simulink model "dof"  (R2024b)
settings: Solver=VariableStepAuto  StartTime=0.0  StopTime=200  RelTol=1e-3
libraries: aerolibanim x1, shared6dof x1, aerolibatmos2 x1, aerolibasang x1
settings Model: Creator=isaac  LastModifiedBy=Isaac

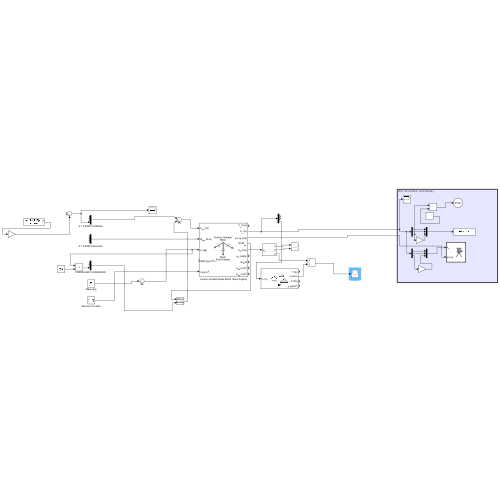
[thumbnail: Simulink's stored preview of the top-level diagram]
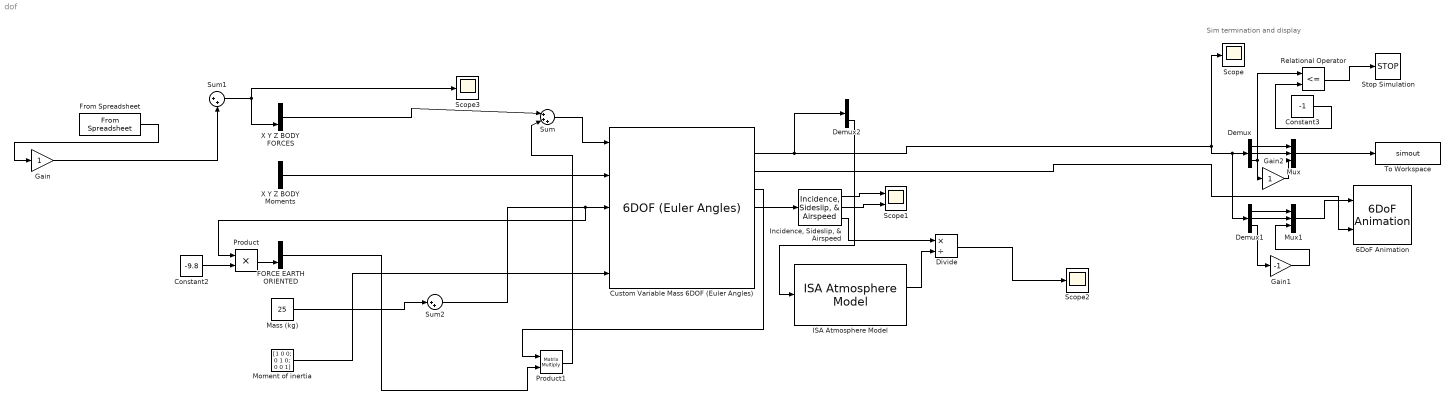
== system dof ==
  note: Sim termination and display
  6DoF Animation : aerolibanim/6DoF Animation  u1=[-5000 5000 -5000 5000 -15000 0]  u2=0.1  u3=50  u4=[4000 0 -5000]  u5=Fly alongside  u6=[20000 5000 -30000]  u7=10  u8=on
  Constant2 : Constant  Value=-9.8
  Constant3 : Constant  Value=-1
  Custom Variable Mass 6DOF (Euler Angles) : shared6dof/6DOF (Euler Angles)  units=Metric (MKS)  mtype=Custom Variable  rep=Euler Angles  xme_0=[0 0 0]  Vm_0=[0 0 0]  eul_0=[0.002 0.001 -0.01]  pm_0=[0.01 0 0]  mass_0=1.0  mass_e=0.5  mass_f=2.0  inertia=eye(3)  inertia_e=eye(3)  inertia_f=2*eye(3)  k_quat=1.0  vre_flag=off  abi_flag=on  aMode=0  xme_statename=''  Vm_statename=''  eul_statename=''  quat_statename=''  pm_statename=''  mass_statename=''
      settings: LibrarySourceBlock=aerolib6dof2/Custom Variable Mass 6DOF (Euler Angles)
  Demux : Demux  Outputs=3
  Demux1 : Demux  Outputs=3
  Demux2 : Demux  Outputs=3
  Divide : Product  Inputs=*/
  FORCE EARTH ORIENTED : Mux  Inputs=3
  From Spreadsheet : FromSpreadsheet  FileName=C:\Users\Isaac\Documents\LERT\Simulations\ncurve.csv  SheetName=ncurve  ExtrapolationAfterLastDataPoint=Hold last value
  Gain : Gain
  Gain1 : Gain  Gain=-1
  Gain2 : Gain
  ISA Atmosphere Model : aerolibatmos2/ISA Atmosphere Model  useExtended=off  action=Warning  custom=off  viscosityOut=off  g=9.80665  gamma=1.4  R=287.0531  L=0.0065  h_trop=11000  h_strat=20000  rho0=1.225  P0=101325  T0=288.15  h0=0  S=110.4  Tref=273.15  muref=1.716e-5
  "Incidence, Sideslip, & Airspeed" : aerolibasang/Incidence, Sideslip, & Airspeed
  Mass (kg) : Constant  Value=25
  Moment of inertia : Constant  Value=[1 0 0; 0 1 0; 0 0 1]
  Mux : Mux  Inputs=3
  Mux1 : Mux  Inputs=3
  Product : Product
  Product1 : Product  Multiplication=Matrix(*)
  Relational Operator : RelationalOperator  Operator=<=  OutDataTypeStr=boolean  RndMeth=Simplest  InputSameDT=off
  Scope : Scope
  Scope1 : Scope  NumInputPorts=2
  Scope2 : Scope
  Scope3 : Scope
  Stop Simulation : Stop
  Sum : Sum  Inputs=|+++
  Sum1 : Sum  Inputs=|++
  Sum2 : Sum  Inputs=|++
  To Workspace : ToWorkspace  VariableName=simout  SaveFormat=Timeseries  SampleTime=-1
  X Y Z BODY FORCES : Mux  Inputs=3
  X Y Z BODY Moments : Mux  Inputs=3
  wires:
  Moment of inertia/1 -> Custom Variable Mass 6DOF (Euler Angles)/5
  Constant2/1 -> Product/2
  Product/1 -> FORCE EARTH ORIENTED/3
  X Y Z BODY FORCES/1 -> Sum/1
  Sum/1 -> Custom Variable Mass 6DOF (Euler Angles)/1
  Product1/1 -> Sum/2
  FORCE EARTH ORIENTED/1 -> Product1/2
  Custom Variable Mass 6DOF (Euler Angles)/2 -> Demux2/1, Demux1/1, Demux/1, Scope/1
  Demux/1 -> Mux/1
  Demux/2 -> Mux/2
  Demux/3 -> Gain2/1, Relational Operator/1
  Gain2/1 -> Mux/3
  Constant3/1 -> Relational Operator/2
  Relational Operator/1 -> Stop Simulation/1
  X Y Z BODY Moments/1 -> Custom Variable Mass 6DOF (Euler Angles)/2
  Custom Variable Mass 6DOF (Euler Angles)/4 -> Product1/1
  Mux/1 -> To Workspace/1
  Demux1/3 -> Gain1/1
  Gain1/1 -> Mux1/3
  Demux1/2 -> Mux1/2
  Demux1/1 -> Mux1/1
  Mux1/1 -> 6DoF Animation/1
  Custom Variable Mass 6DOF (Euler Angles)/3 -> 6DoF Animation/2
  Custom Variable Mass 6DOF (Euler Angles)/5 -> "Incidence, Sideslip, & Airspeed"/1
  "Incidence, Sideslip, & Airspeed"/1 -> Scope1/1
  "Incidence, Sideslip, & Airspeed"/2 -> Scope1/2
  Demux2/3 -> ISA Atmosphere Model/1
  Divide/1 -> Scope2/1
  "Incidence, Sideslip, & Airspeed"/3 -> Divide/1
  ISA Atmosphere Model/2 -> Divide/2
  From Spreadsheet/1 -> Gain/1
  Gain/1 -> Sum1/2
  Sum1/1 -> Scope3/1, X Y Z BODY FORCES/3
  Mass (kg)/1 -> Sum2/1
  Sum2/1 -> Product/1, Custom Variable Mass 6DOF (Euler Angles)/3
